simulink model "Problem_3"  (R2020b)
settings: Solver=VariableStepAuto  StartTime=0.0  StopTime=10.0  RelTol=1e-3
settings Model: Creator=HP  LastModifiedBy=HP

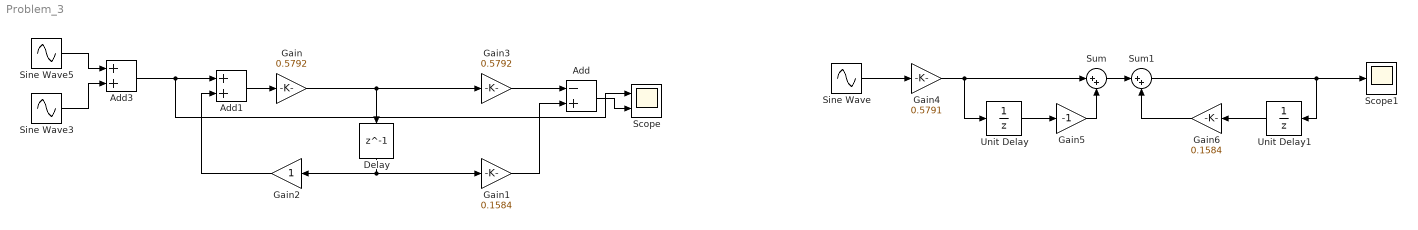
== system Problem_3 ==
  Add : Sum  Inputs=-+
  Add1 : Sum
  Add3 : Sum
  Delay : Delay  DelayLength=1
  Gain : Gain  Gain=0.5792
  Gain1 : Gain  Gain=0.1584
  Gain2 : Gain
  Gain3 : Gain  Gain=0.5792
  Gain4 : Gain  Gain=0.5791
  Gain5 : Gain  Gain=-1
  Gain6 : Gain  Gain=0.1584
  Scope : Scope  NumInputPorts=2
  Scope1 : Scope
  Sine Wave : Sin  SampleTime=0
  Sine Wave3 : Sin  Amplitude=0.5  Frequency=50  SampleTime=0
  Sine Wave5 : Sin  SampleTime=0
  Sum : Sum  Inputs=|++
  Sum1 : Sum  Inputs=|++
  Unit Delay : UnitDelay  SampleTime=-1  HasFrameUpgradeWarning=on
  Unit Delay1 : UnitDelay  SampleTime=-1  HasFrameUpgradeWarning=on
  wires:
  Add3/1 -> Scope/1, Add1/1
  Gain3/1 -> Add/1
  Gain1/1 -> Add/2
  Add/1 -> Scope/2
  Gain/1 -> Delay/1, Gain3/1
  Sine Wave3/1 -> Add3/2
  Gain2/1 -> Add1/2
  Delay/1 -> Gain1/1, Gain2/1
  Sine Wave5/1 -> Add3/1
  Add1/1 -> Gain/1
  Sine Wave/1 -> Gain4/1
  Gain4/1 -> Sum/1, Unit Delay/1
  Unit Delay/1 -> Gain5/1
  Gain5/1 -> Sum/2
  Sum/1 -> Sum1/1
  Gain6/1 -> Sum1/2
  Sum1/1 -> Scope1/1, Unit Delay1/1
  Unit Delay1/1 -> Gain6/1
